simulink model "op_space_robust_control"  (R2019a)
settings: Solver=ode3  StartTime=0.0  StopTime=5  FixedStep=.002  RelTol=1e-3  EnableMultiTasking=on
libraries: simulink x1
settings Model: ExtModeTrigDuration=10000  Creator=smascaro  LastModifiedBy=hoops
settings SolverCC: PositivePriorityOrder=on
settings DataIOCC: SaveFormat=Array  SignalLoggingSaveFormat=ModelDataLogs  SaveOutput=off  SaveTime=off  ReturnWorkspaceOutputs=off
settings OptimizationCC: ExpressionDepthLimit=2147483647  InitFltsAndDblsToZero=on  LifeSpan=inf
settings DebuggingCC: SaveWithParameterizedLinksMsg=none  UnderspecifiedInitializationDetection=Classic  MergeDetectMultiDrivingBlocksExec=none  SignalResolutionControl=TryResolveAllWithWarning  SolverPrmCheckMsg=warning  MultiTaskDSMMsg=warning  MultiTaskCondExecSysMsg=none  FcnCallInpInsideContextMsg=warning  AllowSymbolicDim=off  StateNameClashWarn=warning  SFUnexpectedBacktrackingDiag=warning  SFNoUnconditionalDefaultTransitionDiag=warning  SFExecutionAtInitializationDiag=none  ArithmeticOperatorsInVariantConditions=warning
settings HardwareCC: ProdBitPerPointer=32  ProdBitPerSizeT=32  ProdBitPerPtrDiffT=32  ProdLargestAtomicFloat=None  ProdIntDivRoundTo=Undefined  ProdEndianess=Unspecified  ProdWordSize=32  ProdHWDeviceType=32-bit Generic  TargetBitPerPointer=64  TargetBitPerSizeT=64  TargetBitPerPtrDiffT=64  TargetLongLongMode=on  TargetIntDivRoundTo=Zero  TargetEndianess=LittleEndian  TargetWordSize=64  TargetHWDeviceType=MATLAB Host
settings ModelReferenceCC: PropagateSignalLabelsOutOfModel=off
settings SFSimCC: SimUseLocalCustomCode=off  SimParseCustomCode=off
settings RTWCC: SystemTargetFile=quarc_windows.tlc  TemplateMakefile=quarc_default_tmf  Description=QUARC Win32 Target  RTWUseLocalCustomCode=off
settings CodeAppCC: StateflowObjectComments=on
settings STFCustomTargetCC: TargetPreCompLibLocation=C:\PROGRA~3\QUARC\lib\2015b\windows\release  GeneratePreprocessorConditionals=Disable all  CPPClassGenCompliant=on  SystemTargetFile=quarc_windows.tlc
settings GRTTargetCC: TargetPreCompLibLocation=C:\PROGRA~3\QUARC\lib\2015b\windows\release  TargetLangStandard=C89/C90 (ANSI)  ParMdlRefBuildCompliant=off  CompOptLevelCompliant=off  ConcurrentExecutionCompliant=off  GeneratePreprocessorConditionals=Disable all  CombineOutputUpdateFcns=off  MatFileLogging=off  GRTInterface=on  UseToolchainInfoCompliant=off  ExtMode=on  ExtModeMexFile=quarc_comm
settings ConfigComp: CovMetricSettings=dw  CovHtmlReporting=on  CovSaveCumulativeToWorkspaceVar=on  CovSaveSingleToWorkspaceVar=on  CovExternalEMLEnable=off

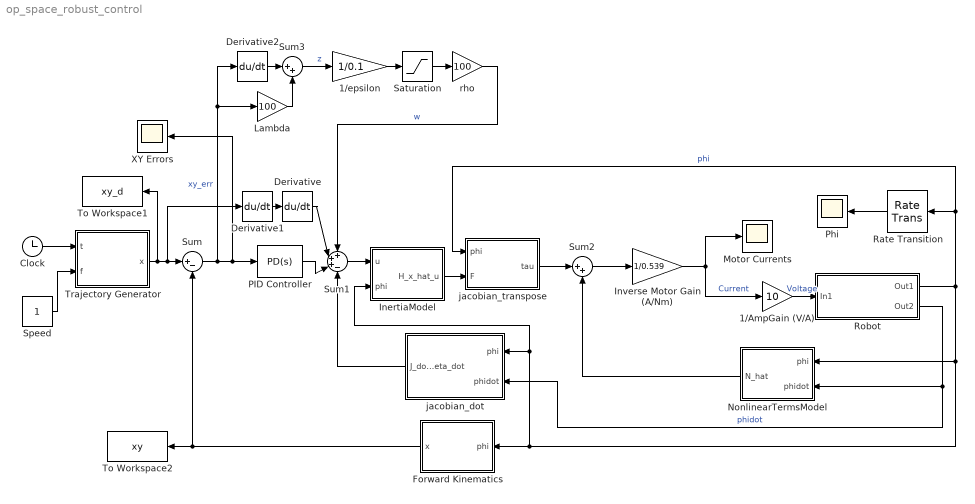
== system op_space_robust_control ==
  1/AmpGain (V/A) : Gain  Gain=10
  1/epsilon : Gain  Gain=1/0.1
  Clock : Clock
  Derivative : Derivative
  Derivative1 : Derivative
  Derivative2 : Derivative
  Forward Kinematics : MATLAB Function  TreatAsAtomicUnit=on
  InertiaModel : MATLAB Function  TreatAsAtomicUnit=on
  Inverse Motor Gain (A/Nm) : Gain  Gain=1/0.539
  Lambda : Gain  Gain=100
  Motor Currents : Scope
  NonlinearTermsModel : MATLAB Function  TreatAsAtomicUnit=on
  PID Controller : simulink/Continuous/PID Controller  Controller=PD  Form=Parallel  TimeDomain=Continuous-time  SampleTime=-1  IntegratorMethod=Forward Euler  FilterMethod=Forward Euler  ControllerParametersSource=internal  P=[1400 1400]  I=1  D=[27 27]  UseFilter=on  N=100  TunerSelectOption=Transfer Function Based (PID Tuner App)  InitialConditionSource=internal  InitialConditionForIntegrator=0  InitialConditionForFilter=0  DifferentiatorICPrevScaledInput=0  ExternalReset=none  TrackingMode=off  Kt=1  LimitOutput=off  UpperSaturationLimit=inf  LowerSaturationLimit=-inf  LinearizeAsGain=on  AntiWindupMode=none  Kb=1  POutMin=[]  POutMax=[]  IOutMin=[]  IOutMax=[]  DOutMin=[]  DOutMax=[]  NOutMin=[]  NOutMax=[]  SumOutMin=[]  SumOutMax=[]  SaturationOutMin=[]  SaturationOutMax=[]  PParamMin=[]  PParamMax=[]  IParamMin=[]  IParamMax=[]  DParamMin=[]  DParamMax=[]  NParamMin=[]  NParamMax=[]  KbParamMin=[]  KbParamMax=[]  KtParamMin=[]  KtParamMax=[]  KbOutMin=[]  KbOutMax=[]  KtOutMin=[]  KtOutMax=[]  IntegratorOutMin=[]  IntegratorOutMax=[]  FilterOutMin=[]  FilterOutMax=[]  SumI1OutMin=[]  SumI1OutMax=[]  SumI2OutMin=[]  SumI2OutMax=[]  SumI3OutMin=[]  SumI3OutMax=[]  SumI4OutMin=[]  SumI4OutMax=[]  SumDOutMin=[]  SumDOutMax=[]  DifferentiatorOutMin=[]  DifferentiatorOutMax=[]  FilterDiffOutCoefMin=[]  FilterDiffOutCoefMax=[]  ReciprocalOutMin=[]  ReciprocalOutMax=[]  SumDenOutMin=[]  SumDenOutMax=[]  SumNumOutMin=[]  SumNumOutMax=[]  DivideOutMin=[]  DivideOutMax=[]  IntegratorContinuousStateAttributes=''  IntegratorStateMustResolveToSignalObject=off  IntegratorRTWStateStorageClass=Auto  FilterContinuousStateAttributes=''  FilterStateMustResolveToSignalObject=off  FilterRTWStateStorageClass=Auto  ParallelPVariant=InternalParameters  IdealPVariant=Disabled  IVariant=Disabled  DVariant=InternalParameters  IntegratorVariant=Disabled  SatVariant=Disabled  AWVariant=Disabled  PCopyVariant=Disabled  TRVariant=Disabled  FdbkBlocksVariant=Forward  IdealPFdbkVariant=Disabled  SatFdbkVariant=Disabled  DerivativeFilterVariant=ContFilter  NVariant=InternalParameters  NCopyVariant=Disabled  FilterICVariant=InternalICsFilter  IntegratorICVariant=Disabled  ExternalResetVariant=Disabled  TRSumVariant=Passthrough  SumFdbkVariant=Disabled  SumVariant=Sum_PD
      settings: AttributesFormatString='PGain='%<P>\n'DGain='%<D>
  Phi : Scope
      settings: AttributesFormatString=SampleTime =%<SampleTime>
  Rate Transition : RateTransition  OutPortSampleTimeOpt=Inherit  OutPortSampleTimeMultiple=10  OutPortSampleTime=0.05
  Robot : Subsystem
      mask Display: disp('Manipulator')
  Saturation : Saturate  UpperLimit=1  LowerLimit=-1
  Speed : Constant
      settings: AttributesFormatString=(circles/sec)
  Sum : Sum  Inputs=|+-
  Sum1 : Sum  Inputs=+++-
  Sum2 : Sum  Inputs=|++
  Sum3 : Sum  Inputs=|++
  To Workspace1 : ToWorkspace  VariableName=xy_d  SampleTime=-1
  To Workspace2 : ToWorkspace  VariableName=xy  SampleTime=-1
  Trajectory Generator : MATLAB Function  TreatAsAtomicUnit=on
  XY Errors : Scope
  jacobian_dot : MATLAB Function  TreatAsAtomicUnit=on
  jacobian_transpose : MATLAB Function  TreatAsAtomicUnit=on
  rho : Gain  Gain=100
  wires:
  Robot/1(Out1) -> NonlinearTermsModel/1(phi), jacobian_dot/1(phi), InertiaModel/2(phi), Forward Kinematics/1(phi), Rate Transition/1, jacobian_transpose/1(phi)  "phi"
  Trajectory Generator/1(x) -> Derivative1/1, Sum/1, To Workspace1/1
  Clock/1 -> Trajectory Generator/1(t)
  Speed/1 -> Trajectory Generator/2(f)
  1/AmpGain (V/A)/1 -> Robot/1(In1)  "Voltage"
  Inverse Motor Gain (A/Nm)/1 -> 1/AmpGain (V/A)/1, Motor Currents/1  "Current"
  Rate Transition/1 -> Phi/1
  Forward Kinematics/1(x) -> To Workspace2/1, Sum/2
  PID Controller/1 -> Sum1/3
  jacobian_transpose/1(tau) -> Sum2/1
  Robot/2(Out2) -> NonlinearTermsModel/2(phidot), jacobian_dot/2(phidot)  "phidot"
  InertiaModel/1(H_x_hat_u) -> jacobian_transpose/2(F)
  Sum1/1 -> InertiaModel/1(u)
  Derivative1/1 -> Derivative/1
  Derivative/1 -> Sum1/2
  Sum2/1 -> Inverse Motor Gain (A/Nm)/1
  NonlinearTermsModel/1(N_hat) -> Sum2/2
  jacobian_dot/1(J_dot_theta_dot) -> Sum1/4
  1/epsilon/1 -> Saturation/1
  Saturation/1 -> rho/1
  rho/1 -> Sum1/1  "w"
  Sum/1 -> Lambda/1, Derivative2/1, PID Controller/1, XY Errors/1  "xy_err"
  Sum3/1 -> 1/epsilon/1  "z"
  Lambda/1 -> Sum3/2
  Derivative2/1 -> Sum3/1

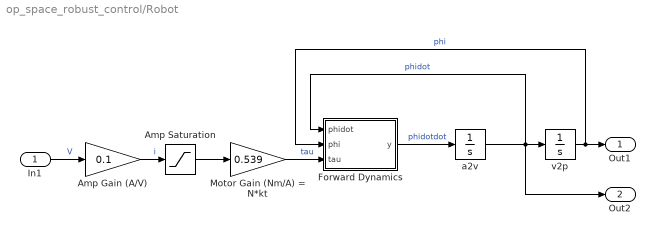
== system op_space_robust_control/Robot ==
  In1 : Inport
  Amp Saturation : Saturate  UpperLimit=1  LowerLimit=-1  ZeroCross=off
  Amp Gain (A/V) : Gain  Gain=0.1
  Forward Dynamics : MATLAB Function  TreatAsAtomicUnit=on
  Motor Gain (Nm/A) = N*kt : Gain  Gain=0.539
  a2v : Integrator
  v2p : Integrator  InitialCondition=[1.1934;-0.2661]
  Out1 : Outport
  Out2 : Outport  Port=2
  wires:
  Forward Dynamics/1(y) -> a2v/1  "phidotdot"
  a2v/1 -> v2p/1, Out2/1, Forward Dynamics/1(phidot)  "phidot"
  v2p/1 -> Out1/1, Forward Dynamics/2(phi)  "phi"
  In1/1 -> Amp Gain (A/V)/1  "V"
  Motor Gain (Nm/A) = N*kt/1 -> Forward Dynamics/3(tau)  "tau"
  Amp Saturation/1 -> Motor Gain (Nm/A) = N*kt/1
  Amp Gain (A/V)/1 -> Amp Saturation/1  "i"

== matlab function op_space_robust_control/jacobian_transpose ==
  data: phi input; F input; tau output
function tau = fcn(phi, F)
% This block supports an embeddable subset of the MATLAB language.
% See the help menu for details. 

a1 = 0.15;  % link 1 length
a2 = 0.15;  % link 2 length
% Describe combined relationship of jacobian from phi to x using jacobian
% (Combines transmission jacobian from phi to theta and manipulator
% jacobian from theta to x)
J11 = -a1*sin(phi(1));
J12 = -a2*sin(phi(2));
J21 = a1*cos(phi(1));
J22 = a2*cos(phi(2));
J = [J11 J12; J21 J22];

tau = transpose(J)*F;

== matlab function op_space_robust_control/Robot/Forward Dynamics ==
  settings: fimath=|
      | fimath(...
      | 'RoundMode', 'floor',...
      | 'OverflowMode', 'wrap',...
      | 'ProductMode', 'KeepLSB', 'ProductWordLength', 32,...
      | 'SumMode', 'KeepLSB', 'SumWordLength', 32,...
      | 'CastBeforeSum', false)
  data: phidot input double size=2; phi input double size=2; y output double size=2; tau input size=2
function y = fcn(phidot,phi,tau)
% This block supports an embeddable subset of the MATLAB language.
% See the help menu for details. 

a1 = 0.15;  % link 1 length
a2 = 0.15;  % link 2 length
m1 = 0.092;  % link 1 mass  
m2 = 0.077; % link 2 mas
r01 = 0.062; % link 1 center of mass
r12 = 0.036; % link 2 COM
I1 = 0.64e-3;  % link 1 inertia
I2 = 0.30e-3;  % link 2 inertia
Jm1 = 0.65e-6; % motor inertias
Jm2 = 0.65e-6;
b1 = 3.1e-6; % viscous damping constants
b2 = 3.1e-6;
c1 = 0.0001; % coulomb friction constants
c2 = 0.0001;
g = 9.8; % gravitational constant
N1 = 70; % gear ratios
N2 = 70;

H11 = N1^2*Jm1 + I1 + m2*a1^2;
H12 = a1*r12*m2*cos(phi(2)-phi(1));
H21 = H12;
H22 = N2^2*Jm2 + I2;
h = a1*r12*m2*sin(phi(2)-phi(1));
G1 = (r01*m1+a1*m2)*g*cos(phi(1));
G2 = r12*m2*g*cos(phi(2));
F1 = N1^2*b1*phidot(1) + N1*c1*sign(phidot(1));
F2 = N2^2*b2*phidot(2) + N2*c2*sign(phidot(2));

H = [H11 H12; H21 H22]; % inertia matrix
V = [0 -h ;h 0]*[phidot(1)^2;phidot(2)^2]; % centripetal torques
G = [G1;G2]; % gravity torques
F = [F1;F2]; % frictional torques

y = inv(H)*(tau - V - G - F); % y=phidotdot

== matlab function op_space_robust_control/InertiaModel ==
  settings: fimath=|
      | fimath(...
      | 'RoundMode', 'floor',...
      | 'OverflowMode', 'wrap',...
      | 'ProductMode', 'KeepLSB', 'ProductWordLength', 32,...
      | 'SumMode', 'KeepLSB', 'SumWordLength', 32,...
      | 'CastBeforeSum', false)
  data: u input double size=2; phi input double size=2; H_x_hat_u output double size=2
function H_x_hat_u = fcn(u,phi)
% This block supports an embeddable subset of the MATLAB language.
% See the help menu for details. 

a1 = 0.15;  % link 1 length
a2 = 0.15;  % link 2 length
m1 = 0.092;  % link 1 mass  
m2 = 0.077; % link 2 mas
r01 = 0.062; % link 1 center of mass
r12 = 0.036; % link 2 COM
I1 = 0.64e-3;  % link 1 inertia
I2 = 0.30e-3;  % link 2 inertia
Jm1 = 0.65e-6; % motor inertias
Jm2 = 0.65e-6;
b1 = 3.1e-6; % viscous damping constants
b2 = 3.1e-6;
c1 = 0.0001; % coulomb friction constants
c2 = 0.0001;
g = 9.8; % gravitational constant
N1 = 70; % gear ratios
N2 = 70;

a1 = 0.15;  % link 1 length
a2 = 0.15;  % link 2 length
% Describe combined relationship of jacobian from phi to x using jacobian
% (Combines transmission jacobian from phi to theta and manipulator
% jacobian from theta to x)
J11 = -a1*sin(phi(1));
J12 = -a2*sin(phi(2));
J21 = a1*cos(phi(1));
J22 = a2*cos(phi(2));
J = [J11 J12; J21 J22];

H11 = N1^2*Jm1 + I1 + m2*a1^2;
H12 = a1*r12*m2*cos(phi(2)-phi(1));
H21 = H12;
H22 = N2^2*Jm2 + I2;

H_hat = [H11 H12; H21 H22]; % inertia matrix

H_x_hat = inv(transpose(J)) * H_hat * inv(J);

H_x_hat_u = H_x_hat * u;

== matlab function op_space_robust_control/Forward Kinematics ==
  settings: fimath=|
      | fimath(...
      | 'RoundMode', 'floor',...
      | 'OverflowMode', 'wrap',...
      | 'ProductMode', 'KeepLSB', 'ProductWordLength', 32,...
      | 'SumMode', 'KeepLSB', 'SumWordLength', 32,...
      | 'CastBeforeSum', false)
  data: x output; phi input
function x = fcn(phi)
% This block supports an embeddable subset of the MATLAB language.
% See the help menu for details. 

a1=0.15;
a2=0.15;
x = [0;0];
x(1) = a1*cos(phi(1))+a2*cos(phi(2));
x(2) = a1*sin(phi(1))+a2*sin(phi(2));

== matlab function op_space_robust_control/NonlinearTermsModel ==
  settings: fimath=|
      | fimath(...
      | 'RoundMode', 'floor',...
      | 'OverflowMode', 'wrap',...
      | 'ProductMode', 'KeepLSB', 'ProductWordLength', 32,...
      | 'SumMode', 'KeepLSB', 'SumWordLength', 32,...
      | 'CastBeforeSum', false)
  data: phi input double size=2; phidot input double size=2; N_hat output double size=2
function N_hat = fcn(phi,phidot)
% This block supports an embeddable subset of the MATLAB language.
% See the help menu for details. 

a1 = 0.15;  % link 1 length
a2 = 0.15;  % link 2 length
m1 = 0.092;  % link 1 mass  
m2 = 0.077; % link 2 mas
r01 = 0.062; % link 1 center of mass
r12 = 0.036; % link 2 COM
I1 = 0.64e-3;  % link 1 inertia
I2 = 0.30e-3;  % link 2 inertia
Jm1 = 0.65e-6; % motor inertias
Jm2 = 0.65e-6;
b1 = 3.1e-6; % viscous damping constants
b2 = 3.1e-6;
c1 = 0.0001; % coulomb friction constants
c2 = 0.0001;
g = 9.8; % gravitational constant
N1 = 70; % gear ratios
N2 = 70;

h = a1*r12*m2*sin(phi(2)-phi(1));
G1 = (r01*m1+a1*m2)*g*cos(phi(1));
G2 = r12*m2*g*cos(phi(2));
F1 = N1^2*b1*phidot(1) + N1*c1*sign(phidot(1));
F2 = N2^2*b2*phidot(2) + N2*c2*sign(phidot(2));

V_hat = [0 -h ;h 0]*[phidot(1)^2;phidot(2)^2]; % centripetal torques
G_hat = [G1;G2]; % gravity torques
F_hat = [F1;F2]; % frictional torques

N_hat = V_hat + G_hat + F_hat;

== matlab function op_space_robust_control/jacobian_dot ==
  data: phi input; J_dot_theta_dot output; phidot input
function J_dot_theta_dot = fcn(phi, phidot)

a1 = 0.15;  % link 1 length
a2 = 0.15;  % link 2 length

J11_dot = -a1*cos(phi(1))*phidot(1);
J12_dot = -a2*cos(phi(2))*phidot(2);
J21_dot = -a1*sin(phi(1))*phidot(1);
J22_dot = -a2*sin(phi(2))*phidot(2);

J_dot = [J11_dot J12_dot; J21_dot J22_dot];

J_dot_theta_dot = J_dot * phidot;

== matlab function op_space_robust_control/Trajectory Generator ==
  settings: fimath=|
      | fimath(...
      | 'RoundMode', 'floor',...
      | 'OverflowMode', 'wrap',...
      | 'ProductMode', 'KeepLSB', 'ProductWordLength', 32,...
      | 'SumMode', 'KeepLSB', 'SumWordLength', 32,...
      | 'CastBeforeSum', false)
  data: x output; t input; f input
function x = fcn(t,f)
% This block supports an embeddable subset of the MATLAB language.
% See the help menu for details. 
x = [0;0];

if t<0.5  % accelerate into circling trajectory
    x(1) = 0.075*cos(2*pi*f*t^2) + 0.125;
    x(2) = 0.075*sin(2*pi*f*t^2) + 0.1;
else  % constant speed circling of radius 0.075 about x=[0.125,0.1]
    x(1) = 0.075*cos(2*pi*f*(t-0.25)) + 0.125;
    x(2) = 0.075*sin(2*pi*f*(t-0.25)) + 0.1;
end
